simulink model "fixed_delays_running_trials"  (R2020b)
settings: Solver=VariableStepAuto  StartTime=0.0  StopTime=100  RelTol=1e-3
libraries: dspspect3 x1
settings Model: Creator=Isabel  LastModifiedBy=Isabel

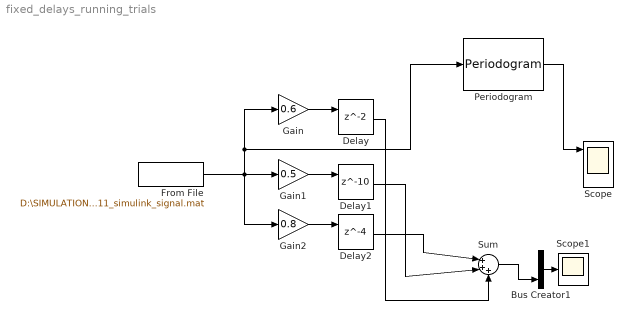
== system fixed_delays_running_trials ==
  Bus Creator1 : BusCreator  Inputs=2
  Delay : Delay  InitialConditionSource=Input port  InitialCondition=0  SampleTime=0.01
      settings: InputPortMap=u0,p4
  Delay1 : Delay  DelayLength=10  InitialConditionSource=Input port  InitialCondition=0  SampleTime=0.01
      settings: InputPortMap=u0,p4
  Delay2 : Delay  DelayLength=4  InitialConditionSource=Input port  InitialCondition=0  SampleTime=0.01
      settings: InputPortMap=u0,p4
  From File : FromFile  FileName=D:\SIMULATIONS_OUTPUT\PAPERS\Model2_3DelayLines_ionChans\UNIFORM\PARAMETERS_RT_period_1us__maxJitter_6simsteps\X11_simulink_signal.mat
  Gain : Gain  Gain=0.6
  Gain1 : Gain  Gain=0.5
  Gain2 : Gain  Gain=0.8
  Periodogram : dspspect3/Periodogram  measurement=Power spectral density  wintype=Hamming  Rs=50  beta=5  winsamp=Symmetric  FFTImplementation=FFTW  inheritFFT=off  fftsize=256  navg=4  inheritTs=on  Ts=1
      settings: SourceProductBaseCode=DS
  Scope : Scope  NumInputPorts=4
  Scope1 : Scope
  Sum : Sum  Inputs=|+++
  wires:
  Sum/1 -> Bus Creator1/2
  Delay2/1 -> Sum/1
  Bus Creator1/1 -> Scope1/1
  Delay1/1 -> Sum/2
  Gain1/1 -> Delay1/1
  Gain/1 -> Delay/1
  From File/1 -> Periodogram/1, Gain/1, Gain2/1, Gain1/1
  Gain2/1 -> Delay2/1
  Delay/1 -> Sum/3
  Periodogram/1 -> Scope/1
